simulink model "NandiniG_23EEM1S02_speedPI"  (R2024b)
settings: Solver=ode3  StartTime=0.0  StopTime=1  FixedStep=1e-6  RelTol=1e-3
libraries: simulink x8, spsVoltageMeasurementLib x6, spsIGBTDiodeLib x6, spsControlledVoltageSourceLib x1, slpidlib x1, spsThreePhaseVIMeasurementLib x1, spspowerguiLib x1
settings Model: Creator=Deepak  LastModifiedBy=INNAGOL2
settings SolverCC: AlgebraicLoopSolver=TrustRegion
settings DebuggingCC: UnconnectedInputMsg=warning  UnconnectedOutputMsg=warning  UnconnectedLineMsg=warning
settings ModelReferenceCC: EnableRefExpFcnMdlSchedulingChecks=on
settings SFSimCC: CustomCodeUndefinedFunction=UseInterfaceOnly
settings RTWCC: GPUComputeCapability=3.5  DLArmComputeVersion=19.05

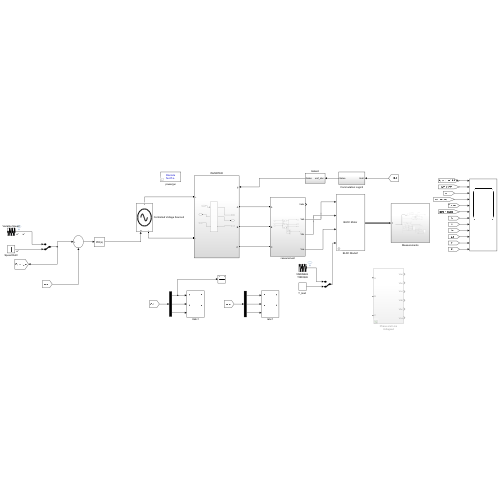
[thumbnail: Simulink's stored preview of the top-level diagram]
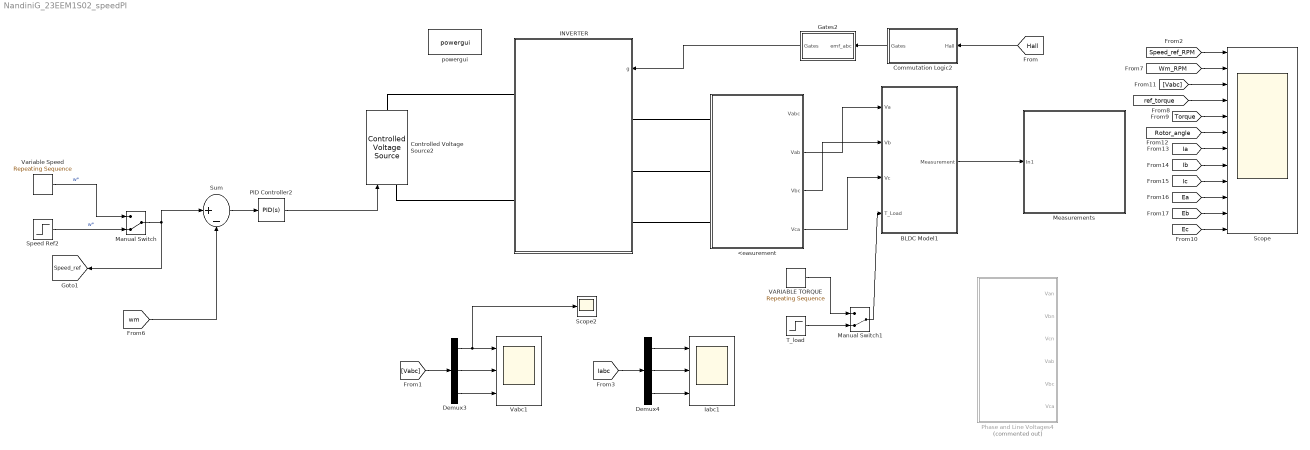
== system NandiniG_23EEM1S02_speedPI ==
  <easurement : Subsystem
  BLDC Model1 : Subsystem  mask(BLDC Motor :){Rs=0.7, Lls=2.7e-3, Phi_m=0.18, J=0.0027, B=0.0004924, P=4}
      mask prompts: Rs "Resistance - Rs [ohms]"; Lls "Inductance - Lls [H]"; Phi_m "Rotor Flux [wb]"; J "Rotor Inertia - J [kg-m^2]"; B "Friction Coefficient -B"; P "No of Poles"
      mask init:
      | Trap=0.5;
      mask Display: fprintf('BLDC Motor')
  Commutation Logic2 : Subsystem
  Controlled Voltage Source2 : spsControlledVoltageSourceLib/Controlled Voltage Source  Initialize=on  Source_Type=DC  Amplitude=160  Phase=0  Frequency=0  Measurements=None
  Demux3 : Demux  Outputs=3
  Demux4 : Demux  Outputs=3
  Gates2 : Subsystem
  INVERTER : Subsystem
  Iabc1 : Scope  NumInputPorts=3
  Manual Switch : ManualSwitch  CurrentSetting=0
  Manual Switch1 : ManualSwitch  CurrentSetting=0
  Measurements : Subsystem
  PID Controller2 : slpidlib/PID Controller  Controller=PID  Form=Parallel  TimeDomain=Continuous-time  UseExternalTs=off  SampleTime=-1  IntegratorMethod=Forward Euler  FilterMethod=Forward Euler  ControllerParametersSource=internal  P=0.01035  I=12.777  UseKiTs=off  D=0  UseExternalDerivativeSource=off  N=0  UseFilter=on  TunerSelectOption=Transfer Function Based (PID Tuner App)  InitialConditionSource=internal  InitialConditionForIntegrator=0  InitialConditionForFilter=0  DifferentiatorICPrevScaledInput=0  ExternalReset=none  TrackingMode=off  Kt=1  LimitOutput=off  SatLimitsSource=internal  UpperSaturationLimit=inf  LowerSaturationLimit=-inf  LinearizeAsGain=on  AntiWindupMode=none  Kb=1  LimitIntegrator=off  UpperIntegratorSaturationLimit=inf  LowerIntegratorSaturationLimit=-inf  POutMin=[]  POutMax=[]  IOutMin=[]  IOutMax=[]  DOutMin=[]  DOutMax=[]  NOutMin=[]  NOutMax=[]  SumOutMin=[]  SumOutMax=[]  SaturationOutMin=[]  SaturationOutMax=[]  PParamMin=[]  PParamMax=[]  IParamMin=[]  IParamMax=[]  DParamMin=[]  DParamMax=[]  NParamMin=[]  NParamMax=[]  KbParamMin=[]  KbParamMax=[]  KtParamMin=[]  KtParamMax=[]  KbOutMin=[]  KbOutMax=[]  KtOutMin=[]  KtOutMax=[]  IntegratorOutMin=[]  IntegratorOutMax=[]  FilterOutMin=[]  FilterOutMax=[]  SumI1OutMin=[]  SumI1OutMax=[]  SumI2OutMin=[]  SumI2OutMax=[]  SumI3OutMin=[]  SumI3OutMax=[]  SumI4OutMin=[]  SumI4OutMax=[]  SumDOutMin=[]  SumDOutMax=[]  DifferentiatorOutMin=[]  DifferentiatorOutMax=[]  FilterDiffOutCoefMin=[]  FilterDiffOutCoefMax=[]  ReciprocalOutMin=[]  ReciprocalOutMax=[]  SumDenOutMin=[]  SumDenOutMax=[]  SumNumOutMin=[]  SumNumOutMax=[]  DivideOutMin=[]  DivideOutMax=[]  UdiffTsProdOutMin=[]  UdiffTsProdOutMax=[]  NTsProdOutMin=[]  NTsProdOutMax=[]  UintegralTsProdOutMin=[]  UintegralTsProdOutMax=[]  UngainTsProdOutMin=[]  UngainTsProdOutMax=[]  ClampingZeroOutDataTypeStr=Inherit: Inherit via back propagation  ClampingZeroOutMin=[]  ClampingZeroOutMax=[]  FilterDenConstantOutDataTypeStr=Inherit: Inherit via back propagation  FilterDenConstantOutMin=[]  FilterDenConstantOutMax=[]  PCopyOutDataTypeStr=Inherit: Inherit via back propagation  PCopyOutMin=[]  PCopyOutMax=[]  NCopyOutDataTypeStr=Inherit: Inherit via back propagation  NCopyOutMin=[]  NCopyOutMax=[]  IntegratorContinuousStateAttributes=''  IntegratorStateMustResolveToSignalObject=off  IntegratorRTWStateStorageClass=Auto  FilterContinuousStateAttributes=''  FilterStateMustResolveToSignalObject=off  FilterRTWStateStorageClass=Auto  ParallelPVariant=InternalParameters  IdealPVariant=Disabled  IVariant=InternalParameters  DVariant=InternalParameters  IntegratorVariant=Continuous  SatVariant=Disabled  AWVariant=Passthrough  PCopyVariant=Disabled  TRVariant=Disabled  FdbkBlocksVariant=Forward  IdealPFdbkVariant=Disabled  SatFdbkVariant=Disabled  DerivativeFilterVariant=ContFilter  NVariant=InternalParameters  NCopyVariant=Disabled  FilterICVariant=InternalICsFilter  IntegratorICVariant=InternalICs  ExternalResetVariant=Disabled  TRSumVariant=Passthrough  SumFdbkVariant=Disabled  SumVariant=Sum_PID  TsampFilterVariant=InternalTs  TsampNgainVariant=Passthrough  TsampIntegralVariant=Disabled_SignalSpec  ExternalSaturationOutDataTypeStr=Inherit: Same as second input  DerivativeSourceVariant=ErrorSignal  PreIntVariant=InternalPreInt
  Phase and Line Voltages4 : Subsystem  Commented=on
  Scope : Scope  NumInputPorts=12
  Scope2 : Scope
  Speed Ref2 : Step  Time=0.1  After=150  SampleTime=0
  Sum : Sum  Inputs=|+-
  "T_load " : Step  Time=0.1  After=5  SampleTime=0
  VARIABLE TORQUE : simulink/Sources/Repeating Sequence  rep_seq_t=[0 1 2 3 4 5 6 7 8 9 10 11 12 13]  rep_seq_y=[3 3 3 3 5 5 5 -2 -2 -2 1 1 1 1 ]
  Vabc1 : Scope  NumInputPorts=3
  Variable Speed : simulink/Sources/Repeating Sequence  rep_seq_t=[0 1 2 3 4 5 6 7 8 9 10 11 11.0001 12 13]  rep_seq_y=[0 20 20 0 0 0 -30 -30 0 0 50 50 40 40 0]
  powergui : spspowerguiLib/powergui  Priority=1  SimulationMode=Discrete  SampleTime=5e-05  frequency=60  Iterations=50  frequencyindice=0  Pbase=100e6  ErrMax=1e-4  UnitsV=kV  UnitsW=MW  buscounter=0  FunctionMessages=off  echomessages=off  EnableUseOfTLC=off  CurrentSourceSwitches=off  DisableSnubberDevices=off  DisableRonSwitches=off  DisableVfSwitches=off  DisplayEquations=off  AutomaticDiscreteSolvers=off  SolverType=Tustin/Backward Euler (TBE)  Interpol=off  ExternalGateDelay=off  methode=off  Ts=100  x0status=blocks  SPID=on  SwTol=0  HookPort=off  NonlinearTolerance=0  nMaxIteration=15  ContinueOnMaxIteration=off  RestoreLinks=warning  ResistiveCurrentMeasurement=off  Frange=[0:2:500]  Ylog=off  Xlog=on  ShowGrid=off  save=off  variable=ZData  structure=0  ZoomFFT=off  StartTime=0.0  cycles=1  DisplayStyle=1  fundamental=60  FreqAxis=off  MaxFrequency=1000  frequencyindicesteady=1  RmsSteady=1  display=off
  tag scope: Speed_ref=global
  wires:
  Sum/1 -> PID Controller2/1
  Commutation Logic2/1(Gates) -> Gates2/1("emf_abc ")
  BLDC Model1/1(Measurement) -> Measurements/1(In1)
  Gates2/1(Gates) -> INVERTER/1(g)
  Manual Switch/1 -> Sum/1, [Speed_ref]
  PID Controller2/1 -> Controlled Voltage Source2/1
  [Wm_RPM] -> Scope/2
  [Ea] -> Scope/10
  [Speed_ref_RPM] -> Scope/1
  [Rotor_angle] -> Scope/6
  [Ec] -> Scope/12
  [Ia] -> Scope/7
  [Torque] -> Scope/5
  [Vabc] -> Scope/3
  [ref_torque] -> Scope/4
  [Ic] -> Scope/9
  [Eb] -> Scope/11
  [Ib] -> Scope/8
  Manual Switch1/1 -> BLDC Model1/4(T_Load)
  VARIABLE TORQUE/1 -> Manual Switch1/1
  "T_load "/1 -> Manual Switch1/2
  Speed Ref2/1 -> Manual Switch/2  "w*"
  Variable Speed/1 -> Manual Switch/1  "w*"
  [Hall] -> Commutation Logic2/1("Hall ")
  [wm] -> Sum/2
  [Iabc] -> Demux4/1
  Demux3/3 -> Vabc1/3
  [Vabc] -> Demux3/1
  Demux3/1 -> Scope2/1, Vabc1/1
  Demux4/1 -> Iabc1/1
  Demux3/2 -> Vabc1/2
  Demux4/2 -> Iabc1/2
  Demux4/3 -> Iabc1/3
  <easurement/2(Vab) -> BLDC Model1/1(Va)
  <easurement/3(Vbc) -> BLDC Model1/2(Vb)
  <easurement/4(Vca) -> BLDC Model1/3(Vc)
  connections:
  Controlled Voltage Source2/RConn1 -- INVERTER/RConn1
  Controlled Voltage Source2/LConn1 -- INVERTER/RConn2
  INVERTER/LConn1 -- <easurement/LConn1
  INVERTER/LConn2 -- <easurement/LConn2
  INVERTER/LConn3 -- <easurement/LConn3

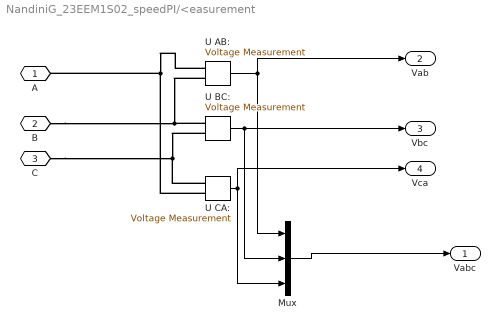
== system NandiniG_23EEM1S02_speedPI/<easurement ==
  Mux : Mux  Inputs=3
  U AB: : spsVoltageMeasurementLib/Voltage Measurement  PhasorSimulation=off  OutputType=Complex  PSBequivalent=0
  U BC: : spsVoltageMeasurementLib/Voltage Measurement  PhasorSimulation=off  OutputType=Complex  PSBequivalent=0
  U CA: : spsVoltageMeasurementLib/Voltage Measurement  PhasorSimulation=off  OutputType=Complex  PSBequivalent=0
  A : PMIOPort  Side=Left
  B : PMIOPort  Port=2  Side=Left
  C : PMIOPort  Port=3  Side=Left
  Vabc : Outport
  Vab : Outport  Port=2
  Vbc : Outport  Port=3
  Vca : Outport  Port=4
  wires:
  U AB:/1 -> Vab/1, Mux/1
  U BC:/1 -> Vbc/1, Mux/2
  U CA:/1 -> Mux/3, Vca/1
  Mux/1 -> Vabc/1
  connections:
  U CA:/LConn1 -- C/RConn1 -- U BC:/LConn2
  U BC:/LConn1 -- U AB:/LConn2 -- B/RConn1
  U AB:/LConn1 -- U CA:/LConn2 -- A/RConn1

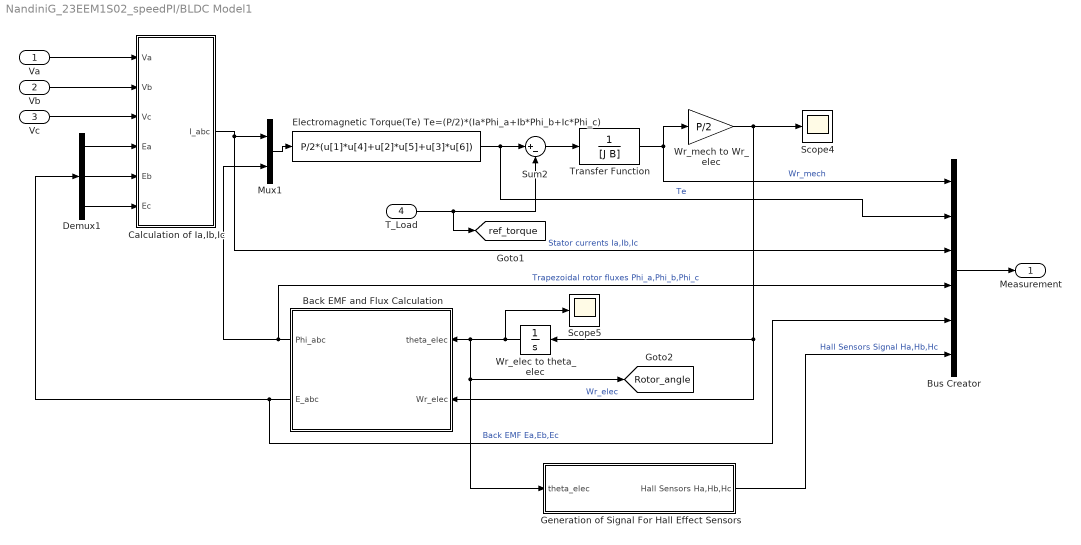
== system NandiniG_23EEM1S02_speedPI/BLDC Model1 ==
  Va : Inport
  Vb : Inport  Port=2
  Vc : Inport  Port=3
  T_Load : Inport  Port=4
  Back EMF and Flux Calculation : Subsystem
  Bus Creator : BusCreator  Inputs=6
  Calculation of Ia,Ib,Ic : Subsystem
  Demux1 : Demux  Outputs=3
  Electromagnetic Torque(Te) Te=(P/2)*(Ia*Phi_a+Ib*Phi_b+Ic*Phi_c) : Fcn  Expr=P/2*(u[1]*u[4]+u[2]*u[5]+u[3]*u[6])
  Generation of Signal For Hall Effect Sensors : Subsystem
  Mux1 : Mux  Inputs=2
  Scope4 : Scope
  Scope5 : Scope
  Sum2 : Sum  Inputs=|+-
  Transfer Function : TransferFcn  Denominator=[J B]
  Wr_elec to theta_elec : Integrator
  Wr_mech to Wr_elec : Gain  Gain=P/2
  Measurement : Outport
  tag scope: Rotor_angle=global, ref_torque=global
  wires:
  Vc/1 -> Calculation of Ia,Ib,Ic/3(Vc)
  Va/1 -> Calculation of Ia,Ib,Ic/1(Va)
  Vb/1 -> Calculation of Ia,Ib,Ic/2(Vb)
  Sum2/1 -> Transfer Function/1
  Mux1/1 -> Electromagnetic Torque(Te) Te=(P/2)*(Ia*Phi_a+Ib*Phi_b+Ic*Phi_c)/1
  Demux1/3 -> Calculation of Ia,Ib,Ic/6(Ec)
  Demux1/2 -> Calculation of Ia,Ib,Ic/5(Eb)
  Demux1/1 -> Calculation of Ia,Ib,Ic/4(Ea)
  Wr_elec to theta_elec/1 -> Generation of Signal For Hall Effect Sensors/1(theta_elec), [Rotor_angle], Back EMF and Flux Calculation/1(theta_elec), Scope5/1
  Bus Creator/1 -> Measurement/1
  Transfer Function/1 -> Wr_mech to Wr_elec/1, Bus Creator/1  "Wr_mech"
  Back EMF and Flux Calculation/2(E_abc) -> Bus Creator/5, Demux1/1  "Back EMF Ea,Eb,Ec"
  Wr_mech to Wr_elec/1 -> Back EMF and Flux Calculation/2(Wr_elec), Wr_elec to theta_elec/1, Scope4/1  "Wr_elec"
  Back EMF and Flux Calculation/1(Phi_abc) -> Mux1/2, Bus Creator/4  "Trapezoidal rotor fluxes Phi_a,Phi_b,Phi_c"
  Calculation of Ia,Ib,Ic/1(I_abc) -> Bus Creator/3, Mux1/1  "Stator currents Ia,Ib,Ic"
  Generation of Signal For Hall Effect Sensors/1(Hall Sensors Ha,Hb,Hc) -> Bus Creator/6  "Hall Sensors Signal Ha,Hb,Hc"
  Electromagnetic Torque(Te) Te=(P/2)*(Ia*Phi_a+Ib*Phi_b+Ic*Phi_c)/1 -> Bus Creator/2, Sum2/1  "Te"
  T_Load/1 -> [ref_torque], Sum2/2

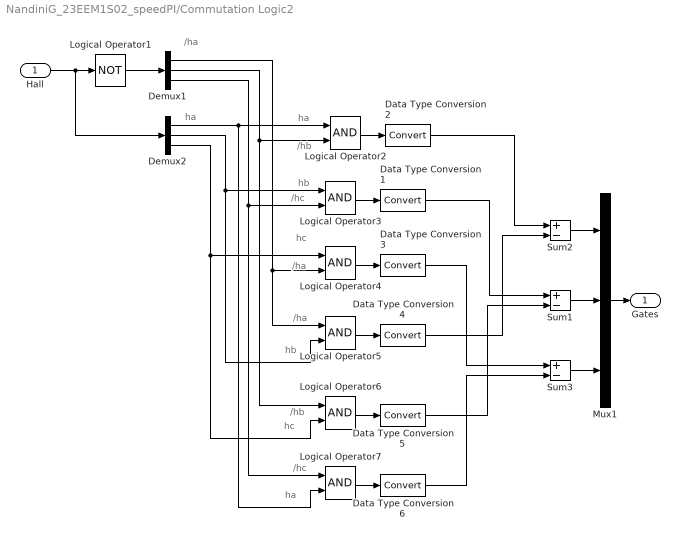
== system NandiniG_23EEM1S02_speedPI/Commutation Logic2 ==
  note: ha
  note: /hc
  note: hc
  note: /hb
  note: hb
  note: /ha
  note: /ha
  note: hc
  note: /hc
  note: hb
  note: /hb
  note: ha
  note: ha
  note: /ha
  "Hall " : Inport
  Data Type Conversion{1..6} (6 alike) : DataTypeConversion  SaturateOnIntegerOverflow=off  RndMeth=Floor
  Demux1 : Demux  Outputs=3
  Demux2 : Demux  Outputs=3
  Logical Operator1 : Logic  Operator=NOT  AllPortsSameDT=off  OutDataTypeStr=boolean
  Logical Operator{2..7} (6 alike) : Logic  AllPortsSameDT=off  OutDataTypeStr=boolean
  Mux1 : Mux  Inputs=3
  Sum1 : Sum  Inputs=+-  OutDataTypeStr=double
  Sum2 : Sum  Inputs=+-  OutDataTypeStr=double
  Sum3 : Sum  Inputs=+-  OutDataTypeStr=double
  Gates : Outport
  wires:
  Demux2/3 -> Logical Operator6/2, Logical Operator4/1
  Sum2/1 -> Mux1/1
  Mux1/1 -> Gates/1
  Logical Operator1/1 -> Demux1/1
  Logical Operator7/1 -> Data Type Conversion6/1
  Sum3/1 -> Mux1/3
  Logical Operator4/1 -> Data Type Conversion3/1
  Data Type Conversion4/1 -> Sum2/2
  Data Type Conversion5/1 -> Sum1/2
  Demux1/1 -> Logical Operator5/1, Logical Operator4/2
  Data Type Conversion3/1 -> Sum3/1
  Data Type Conversion6/1 -> Sum3/2
  Logical Operator5/1 -> Data Type Conversion4/1
  Data Type Conversion2/1 -> Sum2/1
  Logical Operator6/1 -> Data Type Conversion5/1
  Demux1/2 -> Logical Operator2/2, Logical Operator6/1
  Logical Operator2/1 -> Data Type Conversion2/1
  Logical Operator3/1 -> Data Type Conversion1/1
  "Hall "/1 -> Demux2/1, Logical Operator1/1
  Data Type Conversion1/1 -> Sum1/1
  Sum1/1 -> Mux1/2
  Demux2/2 -> Logical Operator5/2, Logical Operator3/1
  Demux1/3 -> Logical Operator3/2, Logical Operator7/1
  Demux2/1 -> Logical Operator2/1, Logical Operator7/2

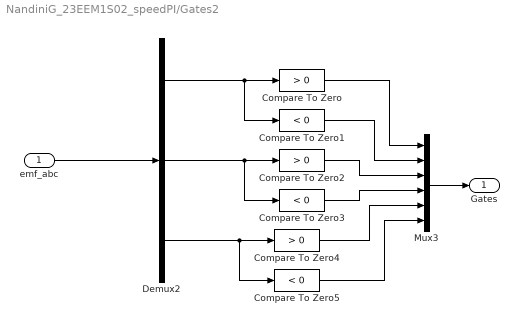
== system NandiniG_23EEM1S02_speedPI/Gates2 ==
  "emf_abc " : Inport
  Compare To Zero : simulink/Logic and Bit Operations/Compare To Zero  relop=>  OutDataTypeStr=boolean  ZeroCross=off
  Compare To Zero1 : simulink/Logic and Bit Operations/Compare To Zero  relop=<  OutDataTypeStr=boolean  ZeroCross=off
  Compare To Zero2 : simulink/Logic and Bit Operations/Compare To Zero  relop=>  OutDataTypeStr=boolean  ZeroCross=off
  Compare To Zero3 : simulink/Logic and Bit Operations/Compare To Zero  relop=<  OutDataTypeStr=boolean  ZeroCross=off
  Compare To Zero4 : simulink/Logic and Bit Operations/Compare To Zero  relop=>  OutDataTypeStr=boolean  ZeroCross=off
  Compare To Zero5 : simulink/Logic and Bit Operations/Compare To Zero  relop=<  OutDataTypeStr=boolean  ZeroCross=off
  Demux2 : Demux  Outputs=3
  Mux3 : Mux  Inputs=6
  Gates : Outport
  wires:
  "emf_abc "/1 -> Demux2/1
  Mux3/1 -> Gates/1
  Demux2/1 -> Compare To Zero/1, Compare To Zero1/1
  Demux2/2 -> Compare To Zero2/1, Compare To Zero3/1
  Demux2/3 -> Compare To Zero4/1, Compare To Zero5/1
  Compare To Zero/1 -> Mux3/1
  Compare To Zero1/1 -> Mux3/2
  Compare To Zero2/1 -> Mux3/3
  Compare To Zero3/1 -> Mux3/4
  Compare To Zero4/1 -> Mux3/5
  Compare To Zero5/1 -> Mux3/6

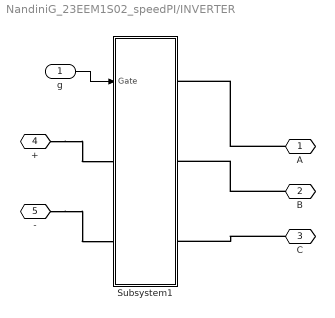
== system NandiniG_23EEM1S02_speedPI/INVERTER ==
  g : Inport
  Subsystem1 : Subsystem
  A : PMIOPort  Side=Left
  B : PMIOPort  Port=2  Side=Left
  C : PMIOPort  Port=3  Side=Left
  + : PMIOPort  Port=4  Side=Right
  - : PMIOPort  Port=5  Side=Right
  wires:
  g/1 -> Subsystem1/1(Gate)
  connections:
  +/RConn1 -- Subsystem1/LConn1
  -/RConn1 -- Subsystem1/LConn2
  C/RConn1 -- Subsystem1/RConn3
  B/RConn1 -- Subsystem1/RConn2
  A/RConn1 -- Subsystem1/RConn1

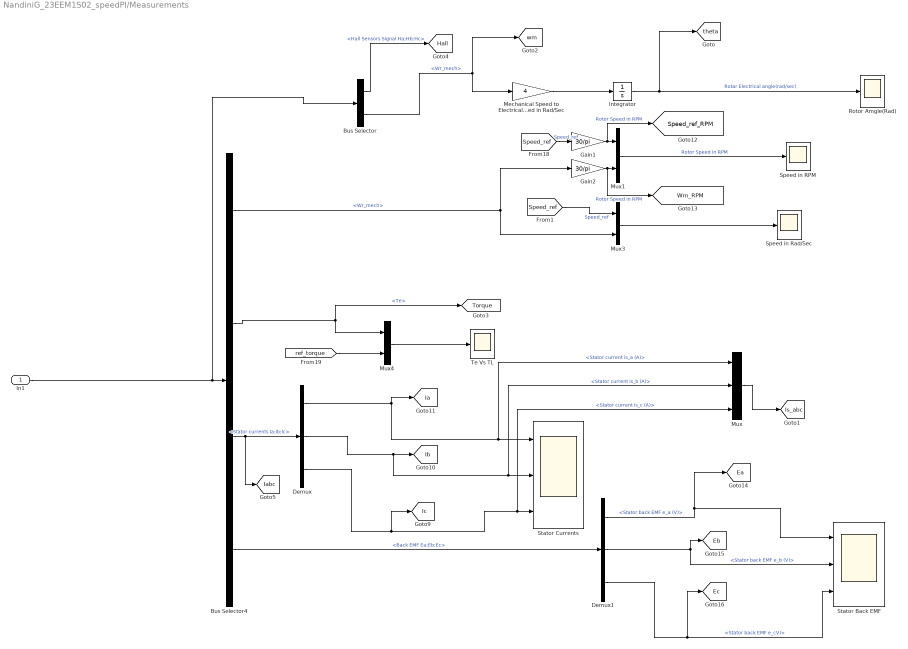
== system NandiniG_23EEM1S02_speedPI/Measurements ==
  In1 : Inport
  Bus Selector : BusSelector  OutputSignals=|
      | Hall Sensors Signal
      | Ha;Hb;Hc,Wr_mech
  Bus Selector4 : BusSelector  OutputSignals=|
      | Wr_mech,Te,Stator currents
      | Ia;Ib;Ic,Back EMF
      | Ea;Eb;Ec
  Demux : Demux  Outputs=3
  Demux1 : Demux  Outputs=3
  Gain1 : Gain  Gain=30/pi
  Gain2 : Gain  Gain=30/pi
  Integrator : Integrator  WrapState=on
  Mechanical Speed to Electrical speed in Rad/Sec : Gain  Gain=4
  Mux : Mux  Inputs=3
  Mux1 : Mux  Inputs=2
  Mux3 : Mux  Inputs=2
  Mux4 : Mux  Inputs=2
  Rotor Amgle(Rad) : Scope
  Speed in RPM : Scope
  Speed in Rad/Sec : Scope
  Stator Back EMF : Scope  NumInputPorts=3
  Stator Currents : Scope  NumInputPorts=3
  Te Vs TL : Scope
  tag scope: Ea=global, Eb=global, Ec=global, Hall=global, Ia=global, Iabc=global, Ib=global, Ic=global, Is_abc=global, Speed_ref_RPM=global, Torque=global, Wm_RPM=global, theta=global, wm=global
  wires:
  [ref_torque] -> Mux4/2
  Mechanical Speed to Electrical speed in Rad/Sec/1 -> Integrator/1
  Mux4/1 -> Te Vs TL/1
  Bus Selector/2 -> Mechanical Speed to Electrical speed in Rad/Sec/1, [wm]  "<Wr_mech>"
  Demux1/2 -> Stator Back EMF/2, [Eb]  "<Stator back EMF e_b (V)>"
  Demux/1 -> Stator Currents/1, Mux/1, [Ia]  "<Stator current is_a (A)>"
  In1/1 -> Bus Selector/1, Bus Selector4/1
  Demux1/3 -> [Ec], Stator Back EMF/3  "<Stator back EMF e_cV)>"
  Gain2/1 -> [Wm_RPM], Mux1/2  "Rotor Speed in RPM"
  Demux/3 -> [Ic], Mux/3, Stator Currents/3  "<Stator current is_c (A)>"
  Integrator/1 -> [theta], Rotor Amgle(Rad)/1  "Rotar Electrical angle(rad/sec)"
  Demux1/1 -> [Ea], Stator Back EMF/1  "<Stator back EMF e_a (V)>"
  Bus Selector4/1 -> Gain2/1, Mux3/2  "<Wr_mech>"
  Gain1/1 -> [Speed_ref_RPM], Mux1/1  "Rotor Speed in RPM"
  Mux3/1 -> Speed in Rad/Sec/1
  Mux1/1 -> Speed in RPM/1  "Rotor Speed in RPM"
  [Speed_ref] -> Gain1/1  "Speed_ref"
  Demux/2 -> Stator Currents/2, Mux/2, [Ib]  "<Stator current is_b (A)>"
  [Speed_ref] -> Mux3/1  "Speed_ref"
  Mux/1 -> [Is_abc]
  Bus Selector/1 -> [Hall]  "<Hall Sensors Signal Ha;Hb;Hc>"
  Bus Selector4/2 -> [Torque], Mux4/1  "<Te>"
  Bus Selector4/3 -> [Iabc], Demux/1  "<Stator currents Ia;Ib;Ic>"
  Bus Selector4/4 -> Demux1/1  "<Back EMF Ea;Eb;Ec>"

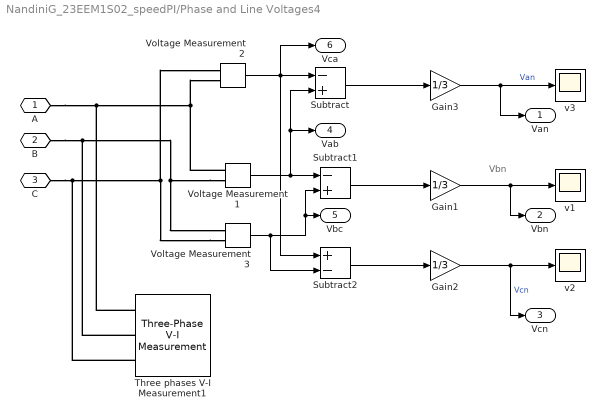
== system NandiniG_23EEM1S02_speedPI/Phase and Line Voltages4 ==
  note: Vbn
  Gain1 : Gain  Gain=1/3
  Gain2 : Gain  Gain=1/3
  Gain3 : Gain  Gain=1/3
  Subtract : Sum  Inputs=-+
  Subtract1 : Sum  Inputs=-+
  Subtract2 : Sum  Inputs=+-
  Three phases V-I Measurement1 : spsThreePhaseVIMeasurementLib/Three-Phase V-I Measurement  VoltageMeasurement=phase-to-phase  SetLabelV=on  LabelV=Vabc  Vpu=off  VpuLL=off  CurrentMeasurement=no  SetLabelI=on  LabelI=Iabc  Ipu=off  Pbase=100e6  Vbase=500e3  OutputType=Complex  PhasorSimulation=off  PSBequivalent=0
  Voltage Measurement1 : spsVoltageMeasurementLib/Voltage Measurement  PhasorSimulation=off  OutputType=Complex  PSBequivalent=0
  Voltage Measurement2 : spsVoltageMeasurementLib/Voltage Measurement  PhasorSimulation=off  OutputType=Complex  PSBequivalent=0
  Voltage Measurement3 : spsVoltageMeasurementLib/Voltage Measurement  PhasorSimulation=off  OutputType=Complex  PSBequivalent=0
  v1 : Scope
  v2 : Scope
  v3 : Scope
  A : PMIOPort  Side=Left
  B : PMIOPort  Port=2  Side=Left
  C : PMIOPort  Port=3  Side=Left
  Van : Outport  VectorParamsAs1DForOutWhenUnconnected=off
  Vbn : Outport  Port=2  VectorParamsAs1DForOutWhenUnconnected=off
  Vcn : Outport  Port=3  VectorParamsAs1DForOutWhenUnconnected=off
  Vab : Outport  Port=4  VectorParamsAs1DForOutWhenUnconnected=off
  Vbc : Outport  Port=5  VectorParamsAs1DForOutWhenUnconnected=off
  Vca : Outport  Port=6  VectorParamsAs1DForOutWhenUnconnected=off
  wires:
  Gain2/1 -> v2/1, Vcn/1  "Vcn"
  Subtract2/1 -> Gain2/1
  Gain1/1 -> v1/1, Vbn/1
  Subtract1/1 -> Gain1/1
  Voltage Measurement3/1 -> Subtract1/2, Vbc/1, Subtract2/2
  Gain3/1 -> v3/1, Van/1  "Van"
  Subtract/1 -> Gain3/1
  Voltage Measurement1/1 -> Vab/1, Subtract/2, Subtract1/1
  Voltage Measurement2/1 -> Vca/1, Subtract2/1, Subtract/1
  connections:
  Voltage Measurement1/LConn1 -- Three phases V-I Measurement1/LConn1 -- A/RConn1 -- Voltage Measurement2/LConn2
  Voltage Measurement1/LConn2 -- Three phases V-I Measurement1/LConn2 -- B/RConn1 -- Voltage Measurement3/LConn1
  Voltage Measurement3/LConn2 -- Three phases V-I Measurement1/LConn3 -- C/RConn1 -- Voltage Measurement2/LConn1

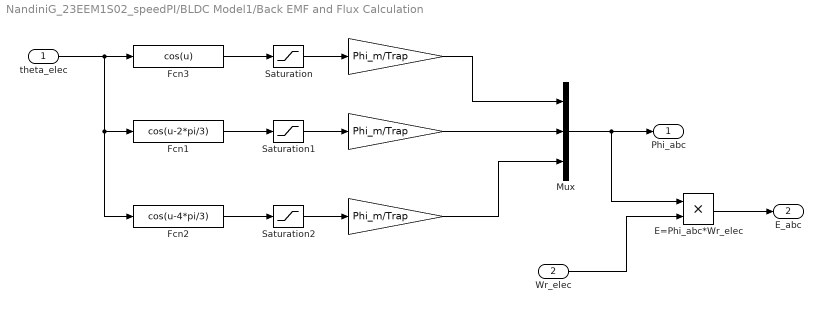
== system NandiniG_23EEM1S02_speedPI/BLDC Model1/Back EMF and Flux Calculation ==
  theta_elec : Inport
  Wr_elec : Inport  Port=2
  " " : Gain  Gain=Phi_m/Trap
  " " : Gain  Gain=Phi_m/Trap
  " " : Gain  Gain=Phi_m/Trap
  E=Phi_abc*Wr_elec : Product
  Fcn1 : Fcn  Expr=cos(u-2*pi/3)
  Fcn2 : Fcn  Expr=cos(u-4*pi/3)
  Fcn3 : Fcn  Expr=cos(u)
  Mux : Mux  Inputs=3
  Saturation : Saturate  UpperLimit=Trap  LowerLimit=-Trap
  Saturation1 : Saturate  UpperLimit=Trap  LowerLimit=-Trap
  Saturation2 : Saturate  UpperLimit=Trap  LowerLimit=-Trap
  Phi_abc : Outport
  E_abc : Outport  Port=2
  wires:
  Fcn3/1 -> Saturation/1
  theta_elec/1 -> Fcn2/1, Fcn1/1, Fcn3/1
  Fcn2/1 -> Saturation2/1
  Fcn1/1 -> Saturation1/1
  " "/1 -> Mux/1
  " "/1 -> Mux/2
  " "/1 -> Mux/3
  Mux/1 -> Phi_abc/1, E=Phi_abc*Wr_elec/1
  Wr_elec/1 -> E=Phi_abc*Wr_elec/2
  E=Phi_abc*Wr_elec/1 -> E_abc/1
  Saturation/1 -> " "/1
  Saturation1/1 -> " "/1
  Saturation2/1 -> " "/1

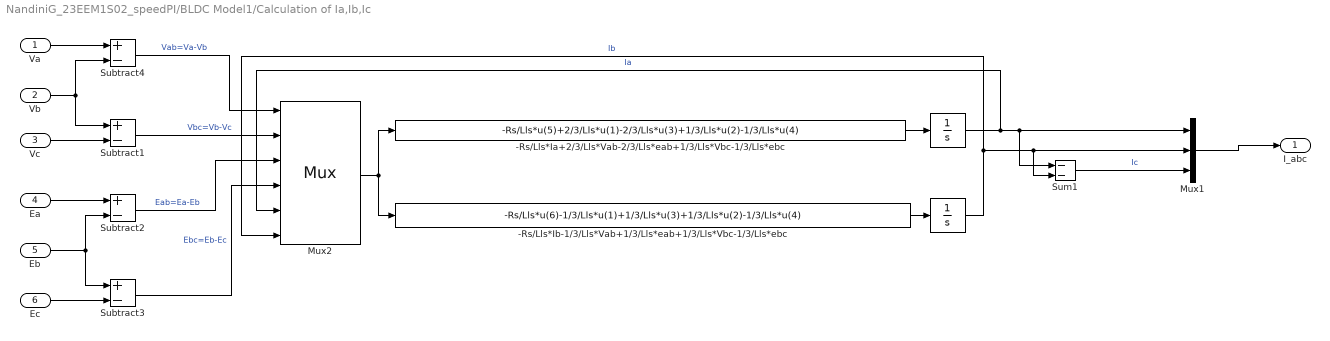
== system NandiniG_23EEM1S02_speedPI/BLDC Model1/Calculation of Ia,Ib,Ic ==
  Va : Inport
  Vb : Inport  Port=2
  Vc : Inport  Port=3
  Ea : Inport  Port=4
  Eb : Inport  Port=5
  Ec : Inport  Port=6
  " " : Integrator
  " " : Integrator
  -Rs/Lls*Ia+2/3/Lls*Vab-2/3/Lls*eab+1/3/Lls*Vbc-1/3/Lls*ebc : Fcn  Expr=-Rs/Lls*u(5)+2/3/Lls*u(1)-2/3/Lls*u(3)+1/3/Lls*u(2)-1/3/Lls*u(4)
  -Rs/Lls*Ib-1/3/Lls*Vab+1/3/Lls*eab+1/3/Lls*Vbc-1/3/Lls*ebc : Fcn  Expr=-Rs/Lls*u(6)-1/3/Lls*u(1)+1/3/Lls*u(3)+1/3/Lls*u(2)-1/3/Lls*u(4)
  Mux1 : Mux  Inputs=3
  Mux2 : Mux  Inputs=6
      settings: DisplayOption=signals
  Subtract{1..4} (4 alike) : Sum  Inputs=+-
  Sum1 : Sum  Inputs=--  SaturateOnIntegerOverflow=on
  I_abc : Outport
  wires:
  Va/1 -> Subtract4/1
  Vb/1 -> Subtract4/2, Subtract1/1
  Vc/1 -> Subtract1/2
  Eb/1 -> Subtract3/1, Subtract2/2
  Ea/1 -> Subtract2/1
  Ec/1 -> Subtract3/2
  -Rs/Lls*Ia+2/3/Lls*Vab-2/3/Lls*eab+1/3/Lls*Vbc-1/3/Lls*ebc/1 -> " "/1
  Subtract3/1 -> Mux2/4  "Ebc=Eb-Ec"
  -Rs/Lls*Ib-1/3/Lls*Vab+1/3/Lls*eab+1/3/Lls*Vbc-1/3/Lls*ebc/1 -> " "/1
  Subtract4/1 -> Mux2/1  "Vab=Va-Vb"
  Subtract1/1 -> Mux2/2  "Vbc=Vb-Vc"
  Subtract2/1 -> Mux2/3  "Eab=Ea-Eb"
  Mux2/1 -> -Rs/Lls*Ia+2/3/Lls*Vab-2/3/Lls*eab+1/3/Lls*Vbc-1/3/Lls*ebc/1, -Rs/Lls*Ib-1/3/Lls*Vab+1/3/Lls*eab+1/3/Lls*Vbc-1/3/Lls*ebc/1
  " "/1 -> Mux1/2, Sum1/2, Mux2/6  "Ib"
  " "/1 -> Sum1/1, Mux1/1, Mux2/5  "Ia"
  Sum1/1 -> Mux1/3  "Ic"
  Mux1/1 -> I_abc/1

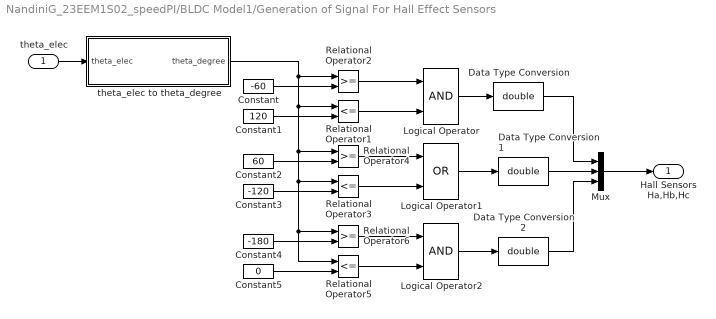
== system NandiniG_23EEM1S02_speedPI/BLDC Model1/Generation of Signal For Hall Effect Sensors ==
  theta_elec : Inport
  Constant : Constant  Value=-60
  Constant1 : Constant  Value=120
  Constant2 : Constant  Value=60
  Constant3 : Constant  Value=-120
  Constant4 : Constant  Value=-180
  Constant5 : Constant  Value=0
  Data Type Conversion : DataTypeConversion  OutDataTypeStr=double
  Data Type Conversion1 : DataTypeConversion  OutDataTypeStr=double
  Data Type Conversion2 : DataTypeConversion  OutDataTypeStr=double
  Logical Operator : Logic  AllPortsSameDT=off  OutDataTypeStr=boolean
  Logical Operator1 : Logic  Operator=OR  AllPortsSameDT=off  OutDataTypeStr=boolean
  Logical Operator2 : Logic  AllPortsSameDT=off  OutDataTypeStr=boolean
  Mux : Mux  Inputs=3
  Relational Operator1 : RelationalOperator  Operator=<=
  Relational Operator2 : RelationalOperator
  Relational Operator3 : RelationalOperator  Operator=<=
  Relational Operator4 : RelationalOperator
  Relational Operator5 : RelationalOperator  Operator=<=
  Relational Operator6 : RelationalOperator
  theta_elec to theta_degree : Subsystem
  Hall Sensors Ha,Hb,Hc : Outport
  wires:
  Constant3/1 -> Relational Operator3/2
  Data Type Conversion2/1 -> Mux/3
  Data Type Conversion1/1 -> Mux/2
  Data Type Conversion/1 -> Mux/1
  Relational Operator5/1 -> Logical Operator2/2
  Logical Operator2/1 -> Data Type Conversion2/1
  Relational Operator6/1 -> Logical Operator2/1
  Constant4/1 -> Relational Operator6/2
  Constant5/1 -> Relational Operator5/2
  Relational Operator3/1 -> Logical Operator1/2
  Logical Operator1/1 -> Data Type Conversion1/1
  Logical Operator/1 -> Data Type Conversion/1
  Mux/1 -> Hall Sensors Ha,Hb,Hc/1
  Relational Operator2/1 -> Logical Operator/1
  Relational Operator1/1 -> Logical Operator/2
  theta_elec to theta_degree/1(theta_degree) -> Relational Operator4/1, Relational Operator3/1, Relational Operator5/1, Relational Operator6/1, Relational Operator1/1, Relational Operator2/1
  Constant/1 -> Relational Operator2/2
  Relational Operator4/1 -> Logical Operator1/1
  Constant1/1 -> Relational Operator1/2
  Constant2/1 -> Relational Operator4/2
  theta_elec/1 -> theta_elec to theta_degree/1(theta_elec)

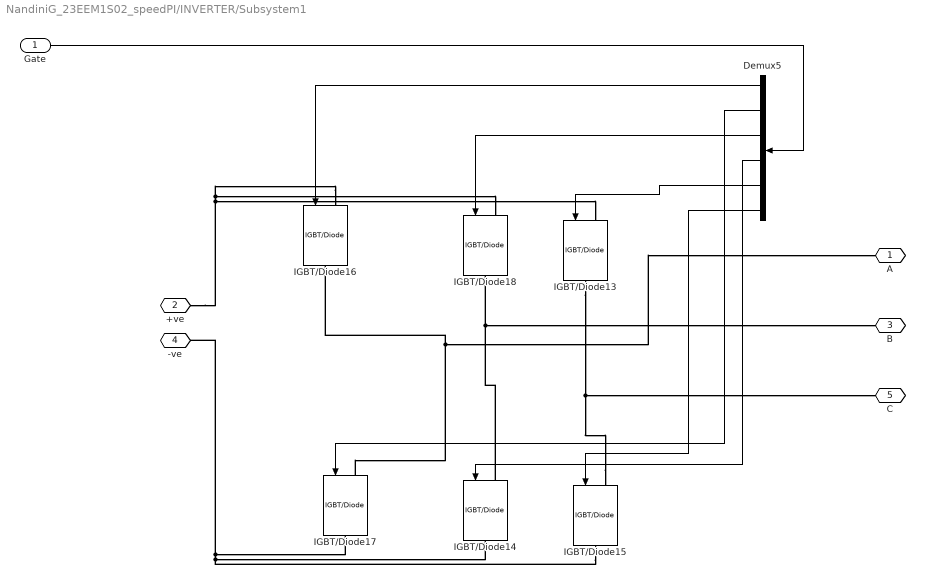
== system NandiniG_23EEM1S02_speedPI/INVERTER/Subsystem1 ==
  Gate : Inport
  Demux5 : Demux  Outputs=6
  IGBT/Diode{13..18} (6 alike) : spsIGBTDiodeLib/IGBT//Diode  Ron=1e-3  Rs=1e5  Cs=inf  Measurements=off
  A : PMIOPort  Side=Right
  +ve : PMIOPort  Port=2  Side=Left
  B : PMIOPort  Port=3  Side=Right
  -ve : PMIOPort  Port=4  Side=Left
  C : PMIOPort  Port=5  Side=Right
  wires:
  Demux5/3 -> IGBT/Diode18/1
  Demux5/2 -> IGBT/Diode17/1
  Demux5/6 -> IGBT/Diode15/1
  Demux5/1 -> IGBT/Diode16/1
  Gate/1 -> Demux5/1
  Demux5/4 -> IGBT/Diode14/1
  Demux5/5 -> IGBT/Diode13/1
  connections:
  IGBT/Diode15/LConn1 -- C/RConn1 -- IGBT/Diode13/RConn1
  IGBT/Diode18/RConn1 -- B/RConn1 -- IGBT/Diode14/LConn1
  IGBT/Diode14/RConn1 -- IGBT/Diode17/RConn1 -- -ve/RConn1 -- IGBT/Diode15/RConn1
  IGBT/Diode16/RConn1 -- A/RConn1 -- IGBT/Diode17/LConn1
  IGBT/Diode16/LConn1 -- IGBT/Diode18/LConn1 -- +ve/RConn1 -- IGBT/Diode13/LConn1

== system NandiniG_23EEM1S02_speedPI/BLDC Model1/Generation of Signal For Hall Effect Sensors/theta_elec to theta_degree ==
  theta_elec : Inport
  Trigonometric Function : Trigonometry
  Trigonometric Function1 : Trigonometry  Operator=cos
  Trigonometric Function2 : Trigonometry  Operator=atan2
  rad to deg : Gain  Gain=180/pi  SaturateOnIntegerOverflow=on  OutDataTypeStr=Inherit: Same as input  ParamDataTypeStr=Inherit: Same as input
  theta_degree : Outport
  wires:
  Trigonometric Function2/1 -> rad to deg/1
  Trigonometric Function/1 -> Trigonometric Function2/1
  Trigonometric Function1/1 -> Trigonometric Function2/2
  theta_elec/1 -> Trigonometric Function1/1, Trigonometric Function/1
  rad to deg/1 -> theta_degree/1
